simulink model "simControlTanque"  (R2020b)
settings: Solver=VariableStepAuto  StartTime=0.0  StopTime=400  RelTol=1e-3
values from neighbouring files (symbols this model uses):
  A = pi    (= 3.14159265359)    [ControlNivel.m]
  h0 = 1.5    [ControlNivel.m]
  Ke = 0.25/10    (= 0.025)    [ControlNivel.m]
  Ks = 0.3543/(10*sqrt(3))    [ControlNivel.m]
  u20 = 5.0    (= 5)    [ControlNivel.m]
libraries: cstblocks x1
settings Model: Creator=bou  LastModifiedBy=bou

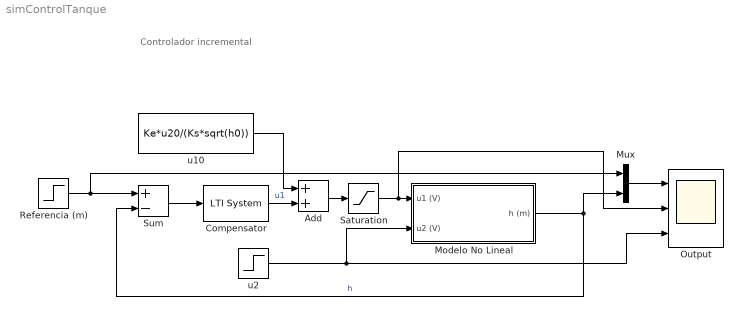
== system simControlTanque ==
  note: Controlador incremental
  Add : Sum
  Compensator : cstblocks/LTI System  sys=C  IC=[]
  Modelo No Lineal : Subsystem
  Mux : Mux  Inputs=2
  Output : Scope  NumInputPorts=3
  Referencia (m) : Step  Time=10  Before=1.5  After=0.25  SampleTime=0
  Saturation : Saturate  UpperLimit=10.0  LowerLimit=0.0
  Sum : Sum  Inputs=+-
  u10 : Constant  Value=Ke*u20/(Ks*sqrt(h0))
  "u2 " : Step  Before=5.0  After=5.0  SampleTime=0
  wires:
  Referencia (m)/1 -> Mux/1, Sum/1
  Sum/1 -> Compensator/1
  Modelo No Lineal/1(h (m)) -> Mux/2, Sum/2  "h"
  "u2 "/1 -> Output/3, Modelo No Lineal/2(u2 (V))
  Compensator/1 -> Add/2  "u1"
  Add/1 -> Saturation/1
  u10/1 -> Add/1
  Mux/1 -> Output/1
  Saturation/1 -> Output/2, Modelo No Lineal/1(u1 (V))

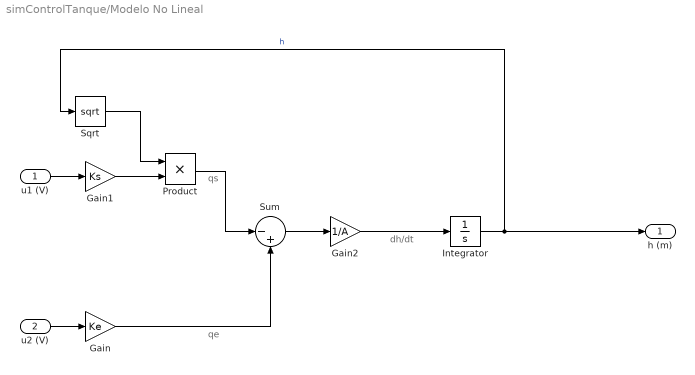
== system simControlTanque/Modelo No Lineal ==
  note: qe
  note: qs
  note: dh/dt
  u1 (V) : Inport
  u2 (V) : Inport  Port=2
  Gain : Gain  Gain=Ke
  Gain1 : Gain  Gain=Ks
  Gain2 : Gain  Gain=1/A
  Integrator : Integrator  InitialCondition=h0
  Product : Product
  Sqrt : Sqrt  SaturateOnIntegerOverflow=on
  Sum : Sum  Inputs=|-+
  h (m) : Outport
  wires:
  Integrator/1 -> h (m)/1, Sqrt/1  "h"
  Gain/1 -> Sum/2
  Gain2/1 -> Integrator/1
  Sqrt/1 -> Product/1
  Sum/1 -> Gain2/1
  u1 (V)/1 -> Gain1/1
  u2 (V)/1 -> Gain/1
  Product/1 -> Sum/1
  Gain1/1 -> Product/2
